simulink model "flexibleMissile"  (R2015a)
settings: Solver=ode45  StartTime=0.0  StopTime=10.0  RelTol=1e-3
values from neighbouring files (symbols this model uses):
  CLd = pi*ARf*Sfins/(1+sqrt(1+(pi*ARf/(2*0.7))^2))/S    [loadModel_EB.m]
  rho = 1.21    [loadModel_EB.m]
  S = pi*D_booster^4/4    (= 0.0131916732161)    [loadModel_EB.m]
  Vx = M*sqrt(gamma_air*r*T)    [loadModel_EB.m]
libraries: RCTblocks x2
settings Model: CovSFcnEnable=off  Creator=s220385  LastModifiedBy=anatole
settings DebuggingCC: SolverPrmCheckMsg=warning

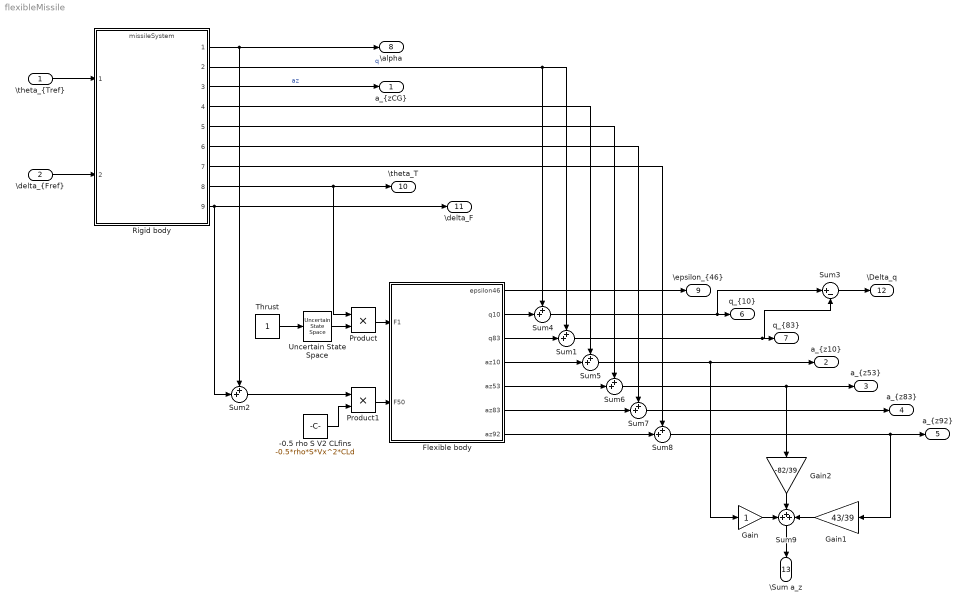
== system flexibleMissile ==
  "\\theta_{Tref}" : Inport
  "\\delta_{Fref}" : Inport  Port=2
  -0.5 rho S V2 CLfins : Constant  Value=-0.5*rho*S*Vx^2*CLd
  Flexible body : Subsystem
      mask Display:
      | port_label('input',1,'Tail Lateral Force')
      | port_label('input',2,'Fins Lateral Force')
      | 
      | port_label('output',1,'\epsilon_{46}','texmode','on')
      | port_label('output',2,'q_{10}','texmode','on')
      | port_label('output',3,'q_{83}','texmode','on')
      | port_label('output',4,'a_{z10}','texmode','on')
      | port_label('output',5,'a_{z53}','texmode','on')
      | port_label('output',6,'a_{z83}','texmode','on')
      | port_label('output',7,'a_{z92}','texmode','on')
  Gain : Gain
  Gain1 : Gain  Gain=43/39
  Gain2 : Gain  Gain=-82/39
  Product : Product
  Product1 : Product
  Rigid body : ModelReference  ModelNameDialog=missileSystem  SimulationMode=Normal  ModelReferenceVersion=1.16  CopyOfModelName=missileSystem  DefaultDataLogging=on
      mask Display:
      | port_label('input',1,'\theta_{Tref}','texmode','on')
      | port_label('input',2,'\delta_{Fref}','texmode','on')
      | 
      | port_label('output',1,'\alpha','texmode','on')
      | port_label('output',2,'q','texmode','on')
      | port_label('output', 3, 'a_{zCG}','texmode','on')
      | port_label('output', 4, 'a_{z10}','texmode','on')
      | port_label('output', 5, 'a_{z53}','texmode','on')
      | port_label('output', 6, 'a_{z83}','texmode','on')
      | port_label('output', 7, 'a_{z91}','texmode','on')
      | port_label('output',8,'\theta_T','texmode','on')
      | port_label('output',9,'\delta_F','texmode','on')
  Sum{1..2,4..8} (7 alike) : Sum  Inputs=++|
  Sum3 : Sum  Inputs=|+-
  Sum9 : Sum  Inputs=+++
  Thrust : Constant
  Uncertain State Space : RCTblocks/Uncertain State Space  Tag=USS  USystem=T0  UValue=[]  X0=[]  uX0=[]
  "a_{zCG}" : Outport
  "a_{z10}" : Outport  Port=2
  "a_{z53}" : Outport  Port=3
  "a_{z83}" : Outport  Port=4
  "a_{z92}" : Outport  Port=5
  "q_{10}" : Outport  Port=6
  "q_{83}" : Outport  Port=7
  \alpha : Outport  Port=8
  "\\epsilon_{46}" : Outport  Port=9
  \theta_T : Outport  Port=10
  \delta_F : Outport  Port=11
  \Delta_q : Outport  Port=12
  \Sum a_z : Outport  Port=13
  wires:
  Product/1 -> Flexible body/1(F1)
  Thrust/1 -> Uncertain State Space/1
  "\\theta_{Tref}"/1 -> Rigid body/1
  Rigid body/1 -> \alpha/1, Sum2/1
  Rigid body/8 -> \theta_T/1, Product/1
  Flexible body/3(q83) -> Sum1/2
  Flexible body/4(az10) -> Sum5/2
  Flexible body/5(az53) -> Sum6/2
  Flexible body/6(az83) -> Sum7/2
  Flexible body/7(az92) -> Sum8/2
  Flexible body/2(q10) -> Sum4/2
  Rigid body/2 -> Sum4/1, Sum1/1  "q"
  Rigid body/4 -> Sum5/1
  Rigid body/5 -> Sum6/1
  Rigid body/6 -> Sum7/1
  Rigid body/7 -> Sum8/1
  Rigid body/3 -> "a_{zCG}"/1  "az"
  Flexible body/1(epsilon46) -> "\\epsilon_{46}"/1
  Sum4/1 -> Sum3/1, "q_{10}"/1
  Sum1/1 -> Sum3/2, "q_{83}"/1
  Sum5/1 -> Gain/1, "a_{z10}"/1
  Sum6/1 -> Gain2/1, "a_{z53}"/1
  Sum7/1 -> "a_{z83}"/1
  Sum8/1 -> Gain1/1, "a_{z92}"/1
  "\\delta_{Fref}"/1 -> Rigid body/2
  Rigid body/9 -> \delta_F/1, Sum2/2
  Sum2/1 -> Product1/1
  Product1/1 -> Flexible body/2(F50)
  -0.5 rho S V2 CLfins/1 -> Product1/2
  Sum3/1 -> \Delta_q/1
  Sum9/1 -> \Sum a_z/1
  Gain/1 -> Sum9/1
  Gain1/1 -> Sum9/3
  Gain2/1 -> Sum9/2
  Uncertain State Space/1 -> Product/2

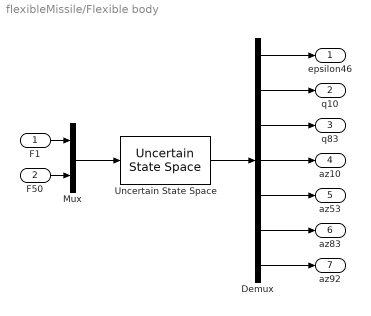
== system flexibleMissile/Flexible body ==
  F1 : Inport
  F50 : Inport  Port=2
  Demux : Demux  Outputs=7
  Mux : Mux  Inputs=2
  Uncertain State Space : RCTblocks/Uncertain State Space  Tag=USS  USystem=flexi  UValue=[]  X0=[]  uX0=[]
  epsilon46 : Outport
  q10 : Outport  Port=2
  q83 : Outport  Port=3
  az10 : Outport  Port=4
  az53 : Outport  Port=5
  az83 : Outport  Port=6
  az92 : Outport  Port=7
  wires:
  Demux/1 -> epsilon46/1
  Demux/2 -> q10/1
  Demux/3 -> q83/1
  Demux/4 -> az10/1
  Demux/5 -> az53/1
  Demux/6 -> az83/1
  Demux/7 -> az92/1
  F1/1 -> Mux/1
  F50/1 -> Mux/2
  Mux/1 -> Uncertain State Space/1
  Uncertain State Space/1 -> Demux/1
